simulink model "Reducer_TestModel"  (R2025a)
settings: Solver=VariableStepAuto  StartTime=0.0  StopTime=100  RelTol=1e-3
PreLoadFcn:
  | defineBus_Rotational
PostLoadFcn:
  | Reducer_TestModelSetup
libraries: fl_lib x22, nesl_utility x9
settings Model: Creator=isaacito  LastModifiedBy=isaacito
settings DataIOCC: DSMLogging=off
settings SimscapeCC: SimscapeLogType=all  SimscapeLogLimitData=off

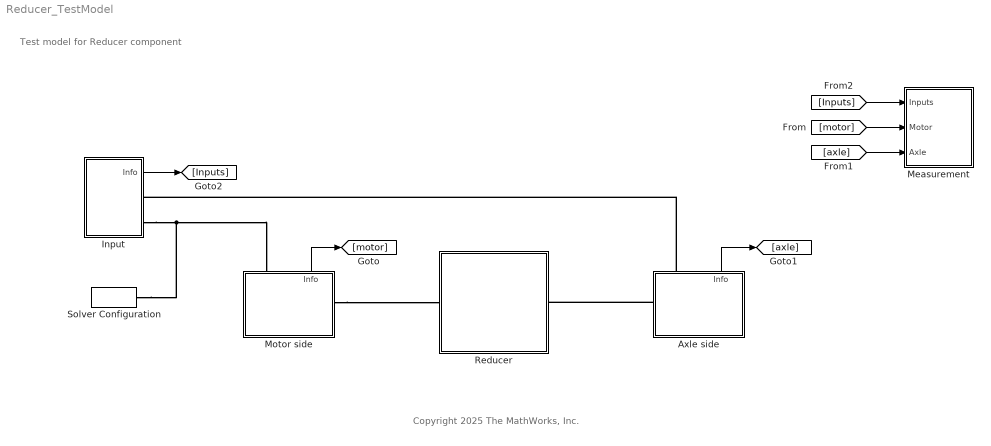
== system Reducer_TestModel ==
  note: Test model for Reducer component
  note: Copyright 2025 The MathWorks, Inc.
  Axle side : Subsystem
      settings: PortSchema="{\"entries\":[{\"content\":{\"sides\":[{\"content\":{\"connectorIds\":[\"LConn1\"]},\"type\":\"ConnectorPlacement.EquallySpacedRectSide\",\"uuid\":\"368d414a-7538-4935-825d-019f7fe99821\"},{\"content\":{\"side\":\"RIGHT\"},\"type\":\"ConnectorPlacement.EquallySpacedRectSide\",\"uuid\":\"14db58ec-4513-4564-8ce5-c8dc0d9cf655\"},{\"content\":{\"connectorIds\":[\"LConn2\",\"Out1\"],\"side\":\"TOP\"},\"type\":\"ConnectorPlacement.EquallySpacedRectSide\",\"uuid\":\"32df8a1b-7de0-4128-b6ae-c4fc856e2ccc\"}]},\"type\":\"ConnectorPlacement.EquallySpacedConnector\",\"uuid\":\"703eb470-82e9-4268-ae65-42db7a05e63d\"}],\"packageUris\":[\"http://schema.mathworks.com/mf0/Connector/R2020b\"],\"version\":\"1.0\"}"
  Input : Subsystem
  Measurement : Subsystem
  Motor side : Subsystem
      settings: PortSchema="{\"entries\":[{\"content\":{\"sides\":[{\"content\":{},\"type\":\"ConnectorPlacement.EquallySpacedRectSide\",\"uuid\":\"368d414a-7538-4935-825d-019f7fe99821\"},{\"content\":{\"connectorIds\":[\"RConn1\"],\"side\":\"RIGHT\"},\"type\":\"ConnectorPlacement.EquallySpacedRectSide\",\"uuid\":\"14db58ec-4513-4564-8ce5-c8dc0d9cf655\"},{\"content\":{\"connectorIds\":[\"LConn1\",\"Out1\"],\"side\":\"TOP\"},\"type\":\"ConnectorPlacement.EquallySpacedRectSide\",\"uuid\":\"32df8a1b-7de0-4128-b6ae-c4fc856e2ccc\"}]},\"type\":\"ConnectorPlacement.EquallySpacedConnector\",\"uuid\":\"703eb470-82e9-4268-ae65-42db7a05e63d\"}],\"packageUris\":[\"http://schema.mathworks.com/mf0/Connector/R2020b\"],\"version\":\"1.0\"}"
  Reducer : Subsystem  ReferencedSubsystem=Reducer_Basic_refsub
  Solver Configuration : nesl_utility/Solver Configuration  PhysicalDomain=network_engine_domain  SubClassName=solver  LeftPortType=input  RightPortType=generic  Tones=[]  Harmonics=[]  SimulateNoise=off  Profile=off  UseLocalSampling=off  EnableSwitchedLinearOptims=on  FrequencyDomain=off  UseCCode=off  RelTol=0.001  AbsTol=0.001  MinStep=1e-09  ToWorkspace=off  RevertToSquareIcSolve=off  NumHomotopyIterations=100  PhasorMode=off  PhasorModeNumHarmonics=1  ConsistencySolver=NEWTON_XTOL_AFTER_FTOL  IndexReductionMethod=DerivativeReplacement  DoDC=off  ResidualTolerance=1e-09  ConsistencyTolSource=GLOBAL  ConsistencyAbsTol=0.001  ConsistencyRelTol=0.001  ConsistencyTolFactor=0.001  UseLocalSolver=off  LocalSolverChoice=NE_BACKWARD_EULER_ADVANCER  ResolveIndetEquations=on  FunctionEvalNumThread=1  LocalSolverSampleTime=0.001  DoFixedCost=off  MaxNonlinIter=3  MaxModeIter=2  ComputeImpulses=off  ImpulseIterations=2  LinearAlgebra=auto  LinearAlgebraNumThread=0  EquationFormulation=NE_TIME_EF  DelaysMemoryBudget=1024  AutomaticFiltering=on  FilteringTimeConstant=0.001  PartitionStorageMethod=AS_NEEDED  PartitionMemoryBudget=1024  PartitionMethod=ROBUST  MultibodyUseLocalSolver=off  MultibodyLocalSolverChoice=ODE1  MultibodyLocalSolverSampleTime=0.001
      settings: AttributesFormatString=Local solver: %<UseLocalSolver>
  wires:
  Motor side/1(Info) -> [motor]
  [motor] -> Measurement/2(Motor)
  [axle] -> Measurement/3(Axle)
  Input/1(Info) -> [Inputs]
  [Inputs] -> Measurement/1(Inputs)
  Axle side/1(Info) -> [axle]
  connections:
  Motor side/RConn1 -- Reducer/LConn1
  Input/RConn2 -- Solver Configuration/RConn1 -- Motor side/LConn1
  Axle side/LConn1 -- Reducer/RConn1
  Axle side/LConn2 -- Input/RConn1

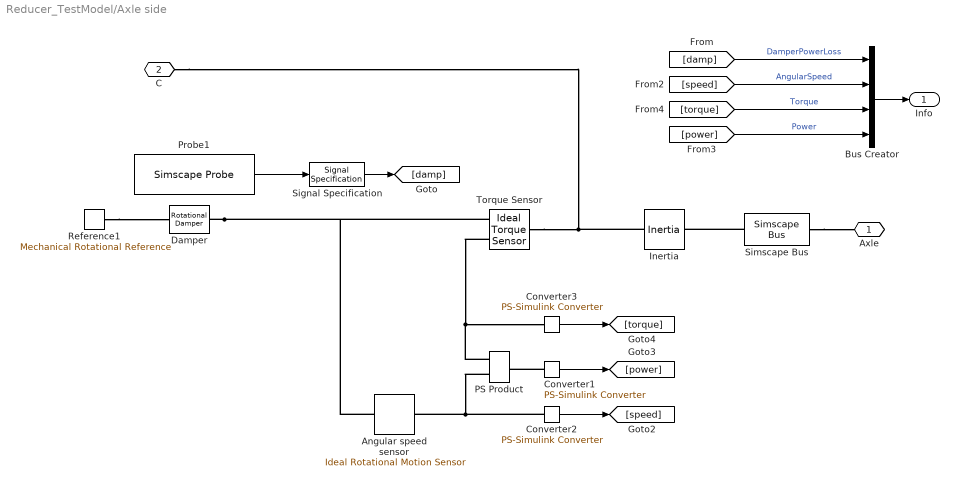
== system Reducer_TestModel/Axle side ==
  Angular speed sensor : fl_lib/Mechanical/Mechanical Sensors/Ideal Rotational Motion Sensor  reference=foundation.enum.MeasurementReference.absolute  acceleration_port=false  velocity_port=true  position_port=false  wrap_angle=false  offset=0 rad
      settings: InternalSimscapePortConfiguration="{\"Bottom\":[],\"Left\":[{\"id\":\"R\",\"label\":\"R\",\"type\":\"foundation.mechanical.rotational.rotational\"}],\"Right\":[{\"id\":\"W\",\"label\":\"W\",\"type\":\"output\"}],\"Top\":[]}"
  Bus Creator : BusCreator  Inputs=4
  Converter1 : nesl_utility/PS-Simulink Converter  PhysicalDomain=network_engine_domain  SubClassName=ps_output  LeftPortType=input  RightPortType=output  PseudoPeriodic=off  Frequencies=[]  VectorFormat=inherit  Unit=W  AffineConversion=off
  Converter2 : nesl_utility/PS-Simulink Converter  PhysicalDomain=network_engine_domain  SubClassName=ps_output  LeftPortType=input  RightPortType=output  PseudoPeriodic=off  Frequencies=[]  VectorFormat=inherit  Unit=rpm  AffineConversion=off
  Converter3 : nesl_utility/PS-Simulink Converter  PhysicalDomain=network_engine_domain  SubClassName=ps_output  LeftPortType=input  RightPortType=output  PseudoPeriodic=off  Frequencies=[]  VectorFormat=inherit  Unit=N*m  AffineConversion=off
  Damper : fl_lib/Mechanical/Rotational Elements/Rotational Damper  D=0.001 N*m*s/rad  w_specify=off  w_priority=None  w=0 rad/s  w_nominal_specify=off  w_nominal_value=1  w_nominal_unit=rad/s  t_specify=off  t_priority=None  t=0 N*m  t_nominal_specify=off  t_nominal_value=1  t_nominal_unit=N*m
      settings: AttributesFormatString=%<D> %<D_unit>
  Inertia : fl_lib/Mechanical/Rotational Elements/Inertia  inertia=1*0.3^2 kg*m^2  num_ports=foundation.enum.numPorts2.two  w_specify=off  w_priority=High  w=0 rad/s  w_nominal_specify=off  w_nominal_value=1  w_nominal_unit=rad/s  t_specify=off  t_priority=None  t=0 N*m  t_nominal_specify=off  t_nominal_value=1  t_nominal_unit=N*m
      settings: AttributesFormatString=%<inertia> %<inertia_unit>  InternalSimscapePortConfiguration="{\"Bottom\":[],\"Left\":[{\"id\":\"I\",\"label\":\"\",\"type\":\"foundation.mechanical.rotational.rotational\"}],\"Right\":[{\"id\":\"J\",\"label\":\"\",\"type\":\"foundation.mechanical.rotational.rotational\"}],\"Top\":[]}"
  PS Product : fl_lib/Physical Signals/Functions/PS Product
  Probe1 : SimscapeProbe  BoundBlock=190  Variables="{\"power_dissipated\":{\"Probing\":\"ON\"},\"t\":{\"Probing\":\"OFF\"},\"w\":{\"Probing\":\"OFF\"}}"
  Reference1 : fl_lib/Mechanical/Rotational Elements/Mechanical Rotational Reference
  Signal Specification : SignalSpecification  Unit=W
  Simscape Bus : SimscapeBus  HierarchyStrings=AngSpd  ConnectionType=Bus: Bus_Rotational
      settings: AttributesFormatString=%<ConnectionType>
  Torque Sensor : fl_lib/Mechanical/Mechanical Sensors/Ideal Torque Sensor
  Axle : PMIOPort  Side=Left
  C : PMIOPort  Port=2  Side=Left
  Info : Outport
  wires:
  Signal Specification/1 -> [damp]
  [power] -> Bus Creator/4  "Power"
  [torque] -> Bus Creator/3  "Torque"
  [speed] -> Bus Creator/2  "AngularSpeed"
  [damp] -> Bus Creator/1  "DamperPowerLoss"
  Converter3/1 -> [torque]
  Converter1/1 -> [power]
  Converter2/1 -> [speed]
  Bus Creator/1 -> Info/1
  Probe1/1 -> Signal Specification/1
  connections:
  PS Product/LConn1 -- Torque Sensor/RConn2 -- Converter3/LConn1
  Damper/LConn1 -- Torque Sensor/RConn1 -- Angular speed sensor/LConn1
  Converter1/LConn1 -- PS Product/RConn1
  PS Product/LConn2 -- Converter2/LConn1 -- Angular speed sensor/RConn1
  Reference1/LConn1 -- Damper/RConn1
  Torque Sensor/LConn1 -- Inertia/RConn1 -- C/RConn1
  Simscape Bus/RConn1 -- Axle/RConn1
  Simscape Bus/LConn1 -- Inertia/LConn1

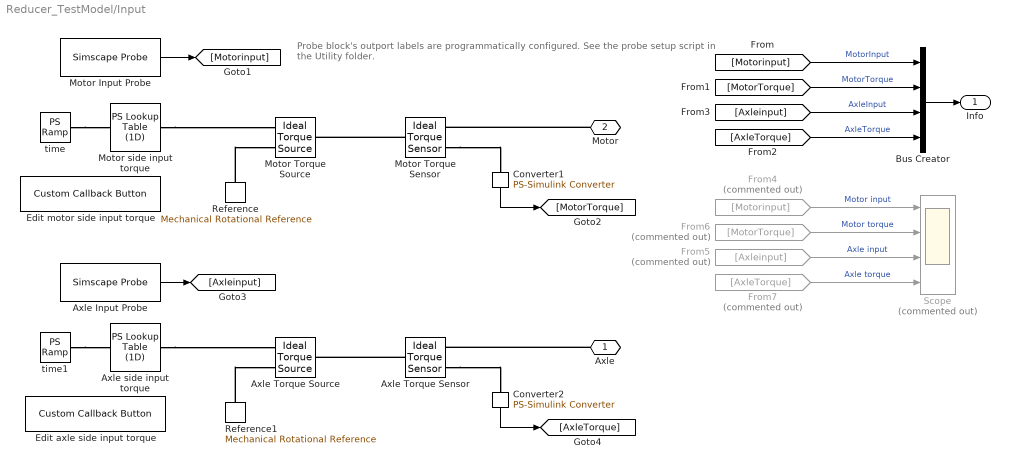
== system Reducer_TestModel/Input ==
  note: Probe block's outport labels are programmatically configured.
      | See the probe setup script in the Utility folder.
  Axle Input Probe : SimscapeProbe  BoundBlock=258  Variables="{\"O\":{\"Unit\":\"N*m\",\"PortLabel\":\"Axle input\",\"Probing\":\"ON\"}}"
  Axle Torque Sensor : fl_lib/Mechanical/Mechanical Sensors/Ideal Torque Sensor
  Axle Torque Source : fl_lib/Mechanical/Mechanical Sources/Ideal Torque Source
  Axle side input torque : fl_lib/Physical Signals/Lookup Tables/PS Lookup Table (1D)  Description=|  x=[0, 1.5, 3, 4, 4.5, 5, 6, 6.5, 7, 8, 9, 10] s  f=[0, 0, 0, -50, -50, -50, 50, 50, 50, 0, 0, 0] N*m  interp_method=simscape.enum.interpolation.smooth  extrap_method=simscape.enum.extrapolation.nearest
      | % This text was automatically inserted by Signal Tool.
      | % SignalDesignMatrixStart
      | [0, 3, 0; 4, 5, -50; 6, 7, 50; 8, 10, 0]
      | % SignalDesignMatrixEnd
  Bus Creator : BusCreator  Inputs=4
  Converter1 : nesl_utility/PS-Simulink Converter  PhysicalDomain=network_engine_domain  SubClassName=ps_output  LeftPortType=input  RightPortType=output  PseudoPeriodic=off  Frequencies=[]  VectorFormat=inherit  Unit=N*m  AffineConversion=off
  Converter2 : nesl_utility/PS-Simulink Converter  PhysicalDomain=network_engine_domain  SubClassName=ps_output  LeftPortType=input  RightPortType=output  PseudoPeriodic=off  Frequencies=[]  VectorFormat=inherit  Unit=N*m  AffineConversion=off
  Edit axle side input torque : CustomCallbackButton  Configuration="{\"components\":[{\"name\":\"BackgroundImageComponent\",\"settings\":{\"image\":{\"size\":[0,0],\"src\":\"default\",\"srcOrientation\":\"Right\"},\"position\":[0,0,1,1]}},{\"name\":\"ButtonStateComponent\",\"settings\":{\"buttonType\":\"momentary\",\"clickFcn\":\"SignalDesignApp(gcs + \\\"\\/Axle side input torque\\\")\",\"onValue\":1,\"position\":[0,0,1,1],\"pressDelay\":\"500\",\"pressFcn\":\"\",\"repeatInterval\":\"0\",\"states\":[{\"horizontalAlignment\":\"center\",\"image\":{\"position\":[0,0,1,1],\"size\":[1,1],\"src\":\"default\",\"srcOrientation\":\"Right\"},\"label\":{\"color\":[0.01176470588,0.01176470588,0.01176470588,1],\"icon\":{\"size\":[0,0],\"src\":\"default\",\"srcOrientation\":\"Right\"},\"iconOffset\":0,\"iconPlacement\":\"left\",\"opacity\":1,\"show\":true,\"text\":{\"content\":\"Signal design app\",\"font\":\"Helvetica\"}},\"labelOffset\":[0,0],\"verticalAlignment\":\"middle\"},{\"horizontalAlignment\":\"center\",\"image\":{\"position\":[0,0,1,1],\"size\":[1,1],\"src\":\"default\",\"srcOrientation\":\"Right\"},\"label\":{\"color\":[0.01176470588,0.01176470588,0.01176470588,1],\"icon\":{\"size\":[0,0],\"src\":\"default\",\"srcOrientation\":\"Right\"},\"iconOffset\":0,\"iconPlacement\":\"left\",\"opacity\":1,\"show\":true,\"text\":{\"content\":\"Signal design app\",\"font\":\"Helvetica\"}},\"labelOffset\":[0,0],\"verticalAlignment\":\"middle\"},{\"horizontalAlignment\":\"center\",\"image\":{\"position\":[0,0,1,1],\"size\":[1,1],\"src\":\"default\",\"srcOrientation\":\"Right\"},\"label\":{\"color\":[0.01176470588,0.01176470588,0.01176470588,1],\"icon\":{\"size\":[0,0],\"src\":\"default\",\"srcOrientation\":\"Right\"},\"iconOffset\":0,\"iconPlacement\":\"left\",\"opacity\":1,\"show\":true,\"text\":{\"content\":\"Signal design app\",\"font\":\"Helvetica\"}},\"labelOffset\":[0,0],\"verticalAlignment\":\"middle\"},{\"horizontalAlignment\":\"center\",\"image\":{\"position\":[0,0,1,1],\"size\":[1,1],\"src\":\"default\",\"srcOrientation\":\"Right\"},\"label\":{\"color\":[0.01176470588,0.01176470588,0.01176470588,1],\"icon\":{\"size\":[0,0],\"src\":\"default\",\"srcOrientation\":\"Right\"},\"iconOffset\":0,\"iconPlacement\":\"left\",\"opacity\":1,\"show\":true,\"text\":{\"content\":\"Signal design app\",\"font\":\"Helvetica\"}},\"labelOffset\":[0,0],\"verticalAlignment\":\"middle\"}]}},{\"name\":\"ForegroundImageComponent\",\"settings\":{\"image\":{\"size\":[0,0],\"src\":\"default\",\"srcOrientation\":\"Right\"},\"isForeground\":1,\"position\":[0,0,1,1]}}],\"derived\":{\"blockParameters\":{\"AutoActivate\":true,\"ButtonText\":\"Signal design app\",\"ButtonType\":\"Momentary\",\"ClickFcn\":\"SignalDesignApp(gcs + \\\"\\/Axle side input torque\\\")\",\"OnValue\":1,\"PressDelay\":\"500\",\"PressFcn\":\"\",\"RepeatInterval\":\"0\",\"fixedAspectRatio\":\"off\"}},\"settings\":{\"BindingType\":\"standalone\",\"autoActivate\":true,\"backgroundColor\":[244,244,244,1],\"backgroundOffset\":0.2,\"backgroundOpacity\":1,\"fixedAspectRatio\":\"off\",\"foregroundColor\":[0.01176470588,0.01176470588,0.01176470588,1],\"migratedFromLegacy\":true,\"useBackgroundColor\":true,\"variant\":\"callback\",\"version\":\"R2025a\"},\"type\":\"Button\"}"  CustomBackgroundColor="{\"color\":[0.9568627451,0.9568627451,0.9568627451],\"show\":true}"
  Edit motor side input torque : CustomCallbackButton  Configuration="{\"components\":[{\"name\":\"BackgroundImageComponent\",\"settings\":{\"image\":{\"size\":[0,0],\"src\":\"default\",\"srcOrientation\":\"Right\"},\"position\":[0,0,1,1]}},{\"name\":\"ButtonStateComponent\",\"settings\":{\"buttonType\":\"momentary\",\"clickFcn\":\"SignalDesignApp(gcs + \\\"\\/Motor side input torque\\\")\",\"onValue\":1,\"position\":[0,0,1,1],\"pressDelay\":\"500\",\"pressFcn\":\"\",\"repeatInterval\":\"0\",\"states\":[{\"horizontalAlignment\":\"center\",\"image\":{\"position\":[0,0,1,1],\"size\":[1,1],\"src\":\"default\",\"srcOrientation\":\"Right\"},\"label\":{\"color\":[0.01176470588,0.01176470588,0.01176470588,1],\"icon\":{\"size\":[0,0],\"src\":\"default\",\"srcOrientation\":\"Right\"},\"iconOffset\":0,\"iconPlacement\":\"left\",\"opacity\":1,\"show\":true,\"text\":{\"content\":\"Signal design app\",\"font\":\"Helvetica\"}},\"labelOffset\":[0,0],\"verticalAlignment\":\"middle\"},{\"horizontalAlignment\":\"center\",\"image\":{\"position\":[0,0,1,1],\"size\":[1,1],\"src\":\"default\",\"srcOrientation\":\"Right\"},\"label\":{\"color\":[0.01176470588,0.01176470588,0.01176470588,1],\"icon\":{\"size\":[0,0],\"src\":\"default\",\"srcOrientation\":\"Right\"},\"iconOffset\":0,\"iconPlacement\":\"left\",\"opacity\":1,\"show\":true,\"text\":{\"content\":\"Signal design app\",\"font\":\"Helvetica\"}},\"labelOffset\":[0,0],\"verticalAlignment\":\"middle\"},{\"horizontalAlignment\":\"center\",\"image\":{\"position\":[0,0,1,1],\"size\":[1,1],\"src\":\"default\",\"srcOrientation\":\"Right\"},\"label\":{\"color\":[0.01176470588,0.01176470588,0.01176470588,1],\"icon\":{\"size\":[0,0],\"src\":\"default\",\"srcOrientation\":\"Right\"},\"iconOffset\":0,\"iconPlacement\":\"left\",\"opacity\":1,\"show\":true,\"text\":{\"content\":\"Signal design app\",\"font\":\"Helvetica\"}},\"labelOffset\":[0,0],\"verticalAlignment\":\"middle\"},{\"horizontalAlignment\":\"center\",\"image\":{\"position\":[0,0,1,1],\"size\":[1,1],\"src\":\"default\",\"srcOrientation\":\"Right\"},\"label\":{\"color\":[0.01176470588,0.01176470588,0.01176470588,1],\"icon\":{\"size\":[0,0],\"src\":\"default\",\"srcOrientation\":\"Right\"},\"iconOffset\":0,\"iconPlacement\":\"left\",\"opacity\":1,\"show\":true,\"text\":{\"content\":\"Signal design app\",\"font\":\"Helvetica\"}},\"labelOffset\":[0,0],\"verticalAlignment\":\"middle\"}]}},{\"name\":\"ForegroundImageComponent\",\"settings\":{\"image\":{\"size\":[0,0],\"src\":\"default\",\"srcOrientation\":\"Right\"},\"isForeground\":1,\"position\":[0,0,1,1]}}],\"derived\":{\"blockParameters\":{\"AutoActivate\":true,\"ButtonText\":\"Signal design app\",\"ButtonType\":\"Momentary\",\"ClickFcn\":\"SignalDesignApp(gcs + \\\"\\/Motor side input torque\\\")\",\"OnValue\":1,\"PressDelay\":\"500\",\"PressFcn\":\"\",\"RepeatInterval\":\"0\",\"fixedAspectRatio\":\"off\"}},\"settings\":{\"BindingType\":\"standalone\",\"autoActivate\":true,\"backgroundColor\":[244,244,244,1],\"backgroundOffset\":0.2,\"backgroundOpacity\":1,\"fixedAspectRatio\":\"off\",\"foregroundColor\":[0.01176470588,0.01176470588,0.01176470588,1],\"migratedFromLegacy\":true,\"useBackgroundColor\":true,\"variant\":\"callback\",\"version\":\"R2025a\"},\"type\":\"Button\"}"  CustomBackgroundColor="{\"color\":[0.9568627451,0.9568627451,0.9568627451],\"show\":true}"
  From4 : From  Commented=on  GotoTag=Motorinput
  From5 : From  Commented=on  GotoTag=Axleinput
  From6 : From  Commented=on  GotoTag=MotorTorque
  From7 : From  Commented=on  GotoTag=AxleTorque
  Motor Input Probe : SimscapeProbe  BoundBlock=254  Variables="{\"O\":{\"Unit\":\"N*m\",\"PortLabel\":\"Motor input\",\"Probing\":\"ON\"}}"
  Motor Torque Sensor : fl_lib/Mechanical/Mechanical Sensors/Ideal Torque Sensor
  Motor Torque Source : fl_lib/Mechanical/Mechanical Sources/Ideal Torque Source
  Motor side input torque : fl_lib/Physical Signals/Lookup Tables/PS Lookup Table (1D)  Description=|  x=[0, 0.5, 1, 4, 17, 30, 40, 45, 50, 60, 70, 80, 90, 95, 100] s  f=[0, 0, 0, 100, 100, 100, 0, 0, 0, -100, -100, -100, 0, 0, 0] N*m  interp_method=simscape.enum.interpolation.smooth  extrap_method=simscape.enum.extrapolation.nearest
      | % This text was automatically inserted by Signal Tool.
      | % SignalDesignMatrixStart
      | [0, 1, 0; 4, 30, 100; 40, 50, 0; 60, 80, -100; 90, 100, 0]
      | % SignalDesignMatrixEnd
  Reference : fl_lib/Mechanical/Rotational Elements/Mechanical Rotational Reference
  Reference1 : fl_lib/Mechanical/Rotational Elements/Mechanical Rotational Reference
  Scope : Scope  Commented=on  NumInputPorts=4
      settings: ActiveDisplayYMinimum=-1  ActiveDisplayYMaximum=1  DataLoggingVariableName=ScopeData2
  time : fl_lib/Physical Signals/Sources/PS Ramp  slope=1  start_time=0 s  initial_output=0 s  ZeroCross=true
  time1 : fl_lib/Physical Signals/Sources/PS Ramp  slope=1  start_time=0 s  initial_output=0 s  ZeroCross=true
  Axle : PMIOPort  Side=Right
  Motor : PMIOPort  Port=2  Side=Right
  Info : Outport
  wires:
  Bus Creator/1 -> Info/1
  Converter1/1 -> [MotorTorque]
  Converter2/1 -> [AxleTorque]
  Axle Input Probe/1 -> [Axleinput]
  [Motorinput] -> Bus Creator/1  "MotorInput"
  [MotorTorque] -> Bus Creator/2  "MotorTorque"
  [Axleinput] -> Bus Creator/3  "AxleInput"
  [AxleTorque] -> Bus Creator/4  "AxleTorque"
  From4/1 -> Scope/1  "Motor input"
  From6/1 -> Scope/2  "Motor torque"
  From5/1 -> Scope/3  "Axle input"
  From7/1 -> Scope/4  "Axle torque"
  Motor Input Probe/1 -> [Motorinput]
  connections:
  Reference/LConn1 -- Motor Torque Source/RConn2
  Motor Torque Sensor/LConn1 -- Motor Torque Source/LConn1
  Motor/RConn1 -- Motor Torque Sensor/RConn1
  Motor Torque Sensor/RConn2 -- Converter1/LConn1
  Axle Torque Sensor/RConn2 -- Converter2/LConn1
  Axle/RConn1 -- Axle Torque Sensor/RConn1
  Axle Torque Sensor/LConn1 -- Axle Torque Source/LConn1
  Axle side input torque/RConn1 -- Axle Torque Source/RConn1
  Reference1/LConn1 -- Axle Torque Source/RConn2
  time/RConn1 -- Motor side input torque/LConn1
  Motor side input torque/RConn1 -- Motor Torque Source/RConn1
  time1/RConn1 -- Axle side input torque/LConn1

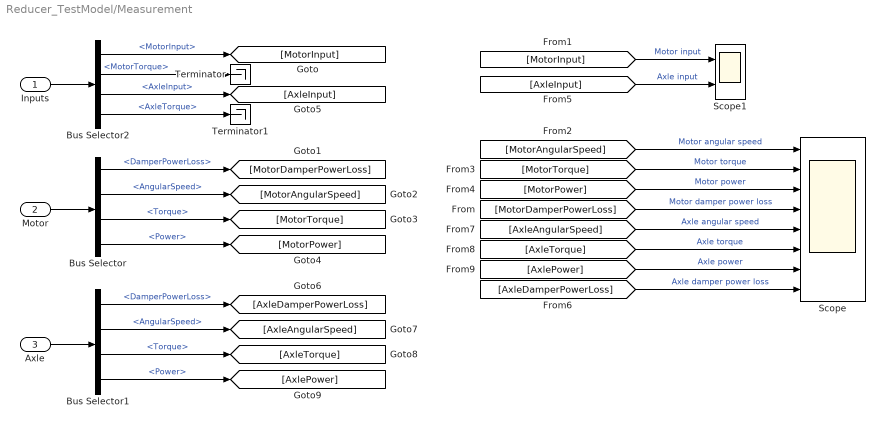
== system Reducer_TestModel/Measurement ==
  Inputs : Inport
  Motor : Inport  Port=2
  Axle : Inport  Port=3
  Bus Selector : BusSelector  OutputSignals=DamperPowerLoss,AngularSpeed,Torque,Power
  Bus Selector1 : BusSelector  OutputSignals=DamperPowerLoss,AngularSpeed,Torque,Power
  Bus Selector2 : BusSelector  OutputSignals=MotorInput,MotorTorque,AxleInput,AxleTorque
  Scope : Scope  NumInputPorts=8
      settings: ActiveDisplayYMinimum=-14777.222667215385  ActiveDisplayYMaximum=32834.961862505406
  Scope1 : Scope  NumInputPorts=2
      settings: ActiveDisplayYMinimum=-1  ActiveDisplayYMaximum=1
  Terminator : Terminator
  Terminator1 : Terminator
  wires:
  Motor/1 -> Bus Selector/1
  Axle/1 -> Bus Selector1/1
  Bus Selector/1 -> [MotorDamperPowerLoss]  "<DamperPowerLoss>"
  Bus Selector/2 -> [MotorAngularSpeed]  "<AngularSpeed>"
  Bus Selector/3 -> [MotorTorque]  "<Torque>"
  Bus Selector/4 -> [MotorPower]  "<Power>"
  Bus Selector1/1 -> [AxleDamperPowerLoss]  "<DamperPowerLoss>"
  Bus Selector1/2 -> [AxleAngularSpeed]  "<AngularSpeed>"
  Bus Selector1/3 -> [AxleTorque]  "<Torque>"
  Bus Selector1/4 -> [AxlePower]  "<Power>"
  Bus Selector2/1 -> [MotorInput]  "<MotorInput>"
  Bus Selector2/3 -> [AxleInput]  "<AxleInput>"
  Bus Selector2/2 -> Terminator/1  "<MotorTorque>"
  Bus Selector2/4 -> Terminator1/1  "<AxleTorque>"
  [MotorInput] -> Scope1/1  "Motor input"
  [AxleInput] -> Scope1/2  "Axle input"
  Inputs/1 -> Bus Selector2/1
  [MotorAngularSpeed] -> Scope/1  "Motor angular speed"
  [MotorTorque] -> Scope/2  "Motor torque"
  [MotorPower] -> Scope/3  "Motor power"
  [MotorDamperPowerLoss] -> Scope/4  "Motor damper power loss"
  [AxleAngularSpeed] -> Scope/5  "Axle angular speed"
  [AxleTorque] -> Scope/6  "Axle torque"
  [AxlePower] -> Scope/7  "Axle power"
  [AxleDamperPowerLoss] -> Scope/8  "Axle damper power loss"

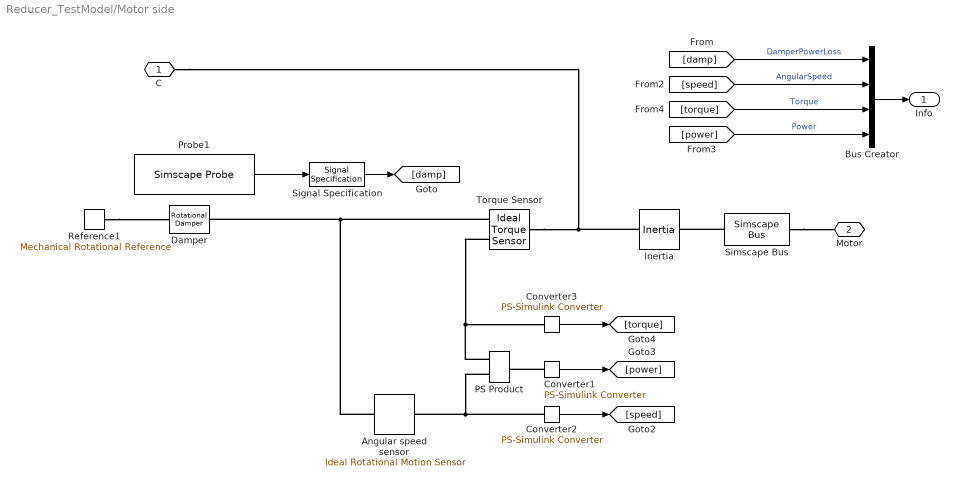
== system Reducer_TestModel/Motor side ==
  Angular speed sensor : fl_lib/Mechanical/Mechanical Sensors/Ideal Rotational Motion Sensor  reference=foundation.enum.MeasurementReference.absolute  acceleration_port=false  velocity_port=true  position_port=false  wrap_angle=false  offset=0 rad
      settings: InternalSimscapePortConfiguration="{\"Bottom\":[],\"Left\":[{\"id\":\"R\",\"label\":\"R\",\"type\":\"foundation.mechanical.rotational.rotational\"}],\"Right\":[{\"id\":\"W\",\"label\":\"W\",\"type\":\"output\"}],\"Top\":[]}"
  Bus Creator : BusCreator  Inputs=4
  Converter1 : nesl_utility/PS-Simulink Converter  PhysicalDomain=network_engine_domain  SubClassName=ps_output  LeftPortType=input  RightPortType=output  PseudoPeriodic=off  Frequencies=[]  VectorFormat=inherit  Unit=W  AffineConversion=off
  Converter2 : nesl_utility/PS-Simulink Converter  PhysicalDomain=network_engine_domain  SubClassName=ps_output  LeftPortType=input  RightPortType=output  PseudoPeriodic=off  Frequencies=[]  VectorFormat=inherit  Unit=rpm  AffineConversion=off
  Converter3 : nesl_utility/PS-Simulink Converter  PhysicalDomain=network_engine_domain  SubClassName=ps_output  LeftPortType=input  RightPortType=output  PseudoPeriodic=off  Frequencies=[]  VectorFormat=inherit  Unit=N*m  AffineConversion=off
  Damper : fl_lib/Mechanical/Rotational Elements/Rotational Damper  D=0.01 N*m*s/rad  w_specify=off  w_priority=None  w=0 rad/s  w_nominal_specify=off  w_nominal_value=1  w_nominal_unit=rad/s  t_specify=off  t_priority=None  t=0 N*m  t_nominal_specify=off  t_nominal_value=1  t_nominal_unit=N*m
      settings: AttributesFormatString=%<D> %<D_unit>
  Inertia : fl_lib/Mechanical/Rotational Elements/Inertia  inertia=10*0.3^2 kg*m^2  num_ports=foundation.enum.numPorts2.two  w_specify=off  w_priority=High  w=0 rad/s  w_nominal_specify=off  w_nominal_value=1  w_nominal_unit=rad/s  t_specify=off  t_priority=None  t=0 N*m  t_nominal_specify=off  t_nominal_value=1  t_nominal_unit=N*m
      settings: AttributesFormatString=%<inertia> %<inertia_unit>  InternalSimscapePortConfiguration="{\"Bottom\":[],\"Left\":[{\"id\":\"I\",\"label\":\"\",\"type\":\"foundation.mechanical.rotational.rotational\"}],\"Right\":[{\"id\":\"J\",\"label\":\"\",\"type\":\"foundation.mechanical.rotational.rotational\"}],\"Top\":[]}"
  PS Product : fl_lib/Physical Signals/Functions/PS Product
  Probe1 : SimscapeProbe  BoundBlock=10  Variables="{\"power_dissipated\":{\"Probing\":\"ON\"},\"t\":{\"Probing\":\"OFF\"},\"w\":{\"Probing\":\"OFF\"}}"
  Reference1 : fl_lib/Mechanical/Rotational Elements/Mechanical Rotational Reference
  Signal Specification : SignalSpecification  Unit=W
  Simscape Bus : SimscapeBus  HierarchyStrings=AngSpd  ConnectionType=Bus: Bus_Rotational
      settings: AttributesFormatString=%<ConnectionType>
  Torque Sensor : fl_lib/Mechanical/Mechanical Sensors/Ideal Torque Sensor
  C : PMIOPort  Side=Left
  Motor : PMIOPort  Port=2  Side=Right
  Info : Outport
  wires:
  Probe1/1 -> Signal Specification/1
  Bus Creator/1 -> Info/1
  Converter2/1 -> [speed]
  Converter1/1 -> [power]
  Converter3/1 -> [torque]
  [damp] -> Bus Creator/1  "DamperPowerLoss"
  [speed] -> Bus Creator/2  "AngularSpeed"
  [torque] -> Bus Creator/3  "Torque"
  [power] -> Bus Creator/4  "Power"
  Signal Specification/1 -> [damp]
  connections:
  Simscape Bus/RConn1 -- Motor/RConn1
  C/RConn1 -- Inertia/RConn1 -- Torque Sensor/LConn1
  Reference1/LConn1 -- Damper/RConn1
  Converter2/LConn1 -- PS Product/LConn2 -- Angular speed sensor/RConn1
  Converter1/LConn1 -- PS Product/RConn1
  Torque Sensor/RConn1 -- Damper/LConn1 -- Angular speed sensor/LConn1
  Torque Sensor/RConn2 -- PS Product/LConn1 -- Converter3/LConn1
  Simscape Bus/LConn1 -- Inertia/LConn1
